simulink model "FBR"  (R2023a)
settings: Solver=VariableStepAuto  StartTime=0.0  StopTime=10/50  RelTol=1e-3
libraries: fl_lib x15, nesl_utility x9
settings Model: Creator=Kaliamoorthy  LastModifiedBy=Kaliamoorthy

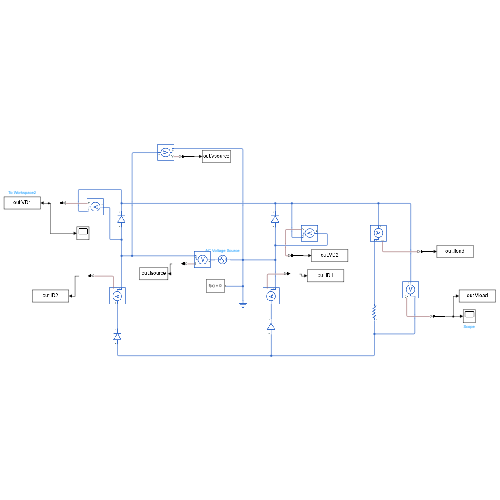
[thumbnail: Simulink's stored preview of the top-level diagram]
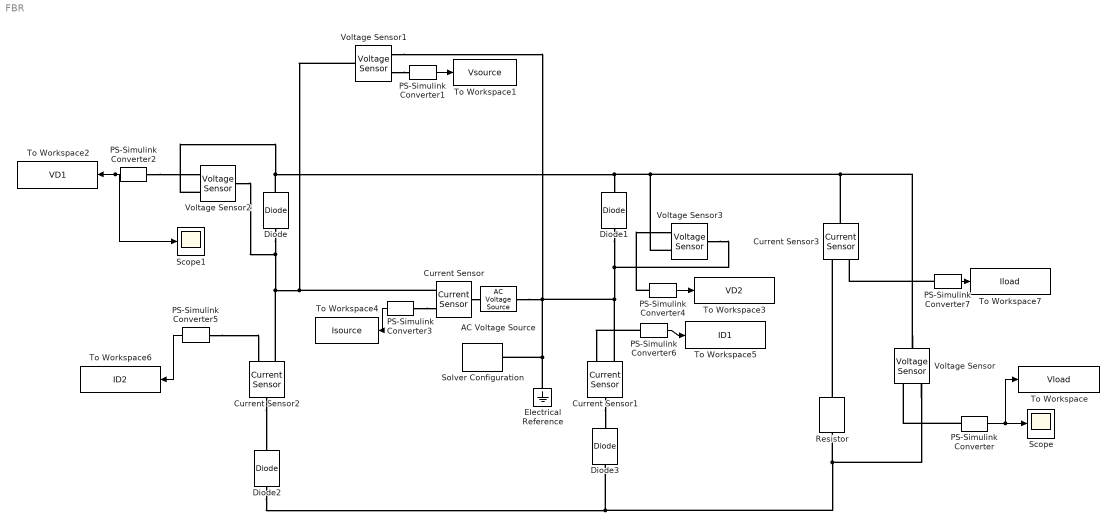
== system FBR ==
  AC Voltage Source : fl_lib/Electrical/Electrical Sources/AC Voltage Source  amp=230*sqrt(2) V  shift=0 deg  frequency=50 Hz  omega=0 rad/s
  Current Sensor{,1..3} (4 alike) : fl_lib/Electrical/Electrical Sensors/Current Sensor
  Diode{,1..3} (4 alike) : fl_lib/Electrical/Electrical Elements/Diode  Vf=0.6 V  Ron=0.3 Ohm  Goff=1e-8 1/Ohm  i_specify=off  i_priority=None  i=0 A  i_nominal_specify=off  i_nominal_unit=A  i_nominal_value=1  v_specify=off  v_priority=None  v=0 V  v_nominal_specify=off  v_nominal_unit=V  v_nominal_value=1
  Electrical Reference : fl_lib/Electrical/Electrical Elements/Electrical Reference
  PS-Simulink Converter{,1..7} (8 alike) : nesl_utility/PS-Simulink Converter  PhysicalDomain=network_engine_domain  SubClassName=ps_output  LeftPortType=input  RightPortType=output  PseudoPeriodic=off  Frequencies=[]  VectorFormat=inherit  Unit=inherit  AffineConversion=off
  Resistor : fl_lib/Electrical/Electrical Elements/Resistor  R=25 Ohm  i_specify=off  i_priority=None  i=0 A  i_nominal_specify=off  i_nominal_unit=A  i_nominal_value=1  v_specify=off  v_priority=None  v=0 V  v_nominal_specify=off  v_nominal_unit=V  v_nominal_value=1
  Scope : Scope
  Scope1 : Scope
  Solver Configuration : nesl_utility/Solver Configuration  PhysicalDomain=network_engine_domain  SubClassName=solver  LeftPortType=input  RightPortType=generic  Tones=[]  Harmonics=[]  SimulateNoise=off  Profile=off  UseLocalSampling=off  EnableSwitchedLinearOptims=on  FrequencyDomain=off  UseCCode=off  RelTol=0.001  AbsTol=0.001  MinStep=1e-09  ToWorkspace=off  RevertToSquareIcSolve=off  NumHomotopyIterations=100  PhasorMode=off  PhasorModeNumHarmonics=1  ConsistencySolver=NEWTON_XTOL_AFTER_FTOL  IndexReductionMethod=DerivativeReplacement  DoDC=off  ResidualTolerance=1e-09  ConsistencyTolSource=GLOBAL  ConsistencyAbsTol=0.001  ConsistencyRelTol=0.001  ConsistencyTolFactor=0.001  UseLocalSolver=on  LocalSolverChoice=NE_BACKWARD_EULER_ADVANCER  ResolveIndetEquations=on  FunctionEvalNumThread=1  LocalSolverSampleTime=5e-5  DoFixedCost=on  MaxNonlinIter=3  MaxModeIter=2  ComputeImpulses=off  ImpulseIterations=2  LinearAlgebra=auto  LinearAlgebraNumThread=0  EquationFormulation=NE_TIME_EF  DelaysMemoryBudget=1024  AutomaticFiltering=on  FilteringTimeConstant=0.001  PartitionStorageMethod=AS_NEEDED  PartitionMemoryBudget=1024  PartitionMethod=ROBUST
  To Workspace : ToWorkspace  VariableName=Vload  SaveFormat=Timeseries  SampleTime=-1
  To Workspace1 : ToWorkspace  VariableName=Vsource  SaveFormat=Timeseries  SampleTime=-1
  To Workspace2 : ToWorkspace  VariableName=VD1  SaveFormat=Timeseries  SampleTime=-1
  To Workspace3 : ToWorkspace  VariableName=VD2  SaveFormat=Timeseries  SampleTime=-1
  To Workspace4 : ToWorkspace  VariableName=Isource  SaveFormat=Timeseries  SampleTime=-1
  To Workspace5 : ToWorkspace  VariableName=ID1  SaveFormat=Timeseries  SampleTime=-1
  To Workspace6 : ToWorkspace  VariableName=ID2  SaveFormat=Timeseries  SampleTime=-1
  To Workspace7 : ToWorkspace  VariableName=Iload  SaveFormat=Timeseries  SampleTime=-1
  Voltage Sensor{,1..3} (4 alike) : fl_lib/Electrical/Electrical Sensors/Voltage Sensor
  wires:
  PS-Simulink Converter/1 -> To Workspace/1, Scope/1
  PS-Simulink Converter1/1 -> To Workspace1/1
  PS-Simulink Converter4/1 -> To Workspace3/1
  PS-Simulink Converter3/1 -> To Workspace4/1
  PS-Simulink Converter6/1 -> To Workspace5/1
  PS-Simulink Converter5/1 -> To Workspace6/1
  PS-Simulink Converter7/1 -> To Workspace7/1
  PS-Simulink Converter2/1 -> Scope1/1, To Workspace2/1
  connections:
  Diode/RConn1 -- Voltage Sensor2/RConn2 -- Voltage Sensor3/RConn2 -- Current Sensor3/LConn1 -- Voltage Sensor/LConn1 -- Diode1/RConn1
  Diode/LConn1 -- Voltage Sensor2/LConn1 -- Voltage Sensor1/LConn1 -- Current Sensor/RConn2 -- Current Sensor2/RConn2
  Electrical Reference/LConn1 -- Diode1/LConn1 -- Voltage Sensor3/LConn1 -- Current Sensor1/RConn2 -- Voltage Sensor1/RConn2 -- AC Voltage Source/RConn1 -- Solver Configuration/RConn1
  PS-Simulink Converter/LConn1 -- Voltage Sensor/RConn1
  Voltage Sensor1/RConn1 -- PS-Simulink Converter1/LConn1
  PS-Simulink Converter2/LConn1 -- Voltage Sensor2/RConn1
  Current Sensor/LConn1 -- AC Voltage Source/LConn1
  Diode2/LConn1 -- Resistor/RConn1 -- Voltage Sensor/RConn2 -- Diode3/LConn1
  PS-Simulink Converter4/LConn1 -- Voltage Sensor3/RConn1
  PS-Simulink Converter3/LConn1 -- Current Sensor/RConn1
  Current Sensor1/LConn1 -- Diode3/RConn1
  Current Sensor2/LConn1 -- Diode2/RConn1
  PS-Simulink Converter5/LConn1 -- Current Sensor2/RConn1
  PS-Simulink Converter6/LConn1 -- Current Sensor1/RConn1
  Resistor/LConn1 -- Current Sensor3/RConn2
  PS-Simulink Converter7/LConn1 -- Current Sensor3/RConn1
